simulink model "controlAerobi"  (R2017b)
settings: Solver=FixedStepDiscrete  StartTime=0.0  StopTime=inf  FixedStep=Ts  RelTol=1e-3
InitFcn:
  | load Navio2_bus;
  | Ts=0.0025;
StopFcn:
  | %save_system('controlAerobi.slx');
  | %run('D:\Eclipse_Workspaces\workspace_rasp\AutoPilot\contAerobi\UpdateFiles\CopyBuildFiles.m');
undefined symbols (not defined in the file or in its folder): DiscIntNeverNeededParam
libraries: simulink x36, sharedutil x1, sharedtransform x1, dspsigops x1
(part 4 of 4)

== matlab function controlAerobi/Sensors/position/px4fow/Liner Fixed-gain Filter1 ==
  data: thrust input; dx input; dy input; quality input; roll input; pitch input; yaw input; a_b input; vx output; vy output; ax output; ay output
function [vx,vy,ax,ay] = linear_Fixed_Gain_Filter(thrust,dx,dy,quality,roll,pitch,yaw,a_b)

dt = 0.0025;
m = 2.5;
mu = 0.87;
R_yaw = [cos(yaw) -sin(yaw);sin(yaw) cos(yaw)];
a_b = a_b/norm(a_b);
a_I = [a_b(2)-sin(pitch);
       -(a_b(1)+sin(roll)*cos(pitch));
       a_b(3)-cos(roll)*cos(pitch)];
persistent x_k P_k
if isempty(x_k)||isempty(P_k)
    x_k = [0;0];
    P_k = [1 0;0 1;];
   
else
%     if thrust < 40
%         thrust = 40;
%     elseif thrust >120
%         thrust = 120;
%     end
%     u = 62.5/thrust;
      
    x_I = [dx;dy];
    
    F = [mu/m          0;
                0   mu/m];
    
    H = [mu/m          0; 
                0   mu/m; 
                1          0;
                0          1;];
            
    Q = diag([1 1]);
    if quality >= 100
        R = diag([0.5 0.5 0.1 0.1]);
    else
        R = diag([0.5 0.5 100000 100000]);
    end
    
    z_k = [a_I(1);a_I(2);x_I(1);x_I(2)];
    y_k = x_k;
        %---------PREDICTION---------%
    %1. Project the state ahead
        x_k = F * x_k;% + B * w_k;
    %2. Project the error covariance ahead
        P_k = F * P_k * F' + Q;  
    %--------CORRECTION----------%
    %1. Compute the Kalman Gain
        K_k = P_k * H' / (H*P_k*H' + R);
        
        resid = z_k - H*y_k;
    %2. Update the estimate via measurement
        x_k = x_k + K_k * resid;
    %3. Update the error covariance
        P_k = (eye(size(K_k,1)) - K_k * H) * P_k;    
    
 
end
v = R_yaw'*x_k;
vx = v(1);
vy = v(2);
ax = a_I(1);
ay = a_I(2);

== matlab function controlAerobi/Sensors/position/EKF_total_Station_Lidar/filter/EKF2_XYZ ==
  data: x_hat output; y_hat output; z_hat output; x input; y input; z input; dx input; dy input; roll input; pitch input; yaw input; acc_ input; d_sf11 input; KQ input; KR input; a_b input; dx_hat output; dy_hat output; dz_hat output
function [x_hat,y_hat,z_hat,dx_hat,dy_hat,dz_hat] = EKF(x,y,z,dx,dy,roll,pitch,yaw,acc_,d_sf11,KQ,KR,a_b)

dt = 0.0025;
a_b = a_b/norm(a_b);
a_I = [(acc_(2)-sin(pitch))*cos(yaw)-sin(yaw)*((-acc_(1)-sin(roll)*cos(pitch)));
        sin(yaw)*(acc_(2)-sin(pitch))+cos(yaw)*((-acc_(1)-sin(roll)*cos(pitch)));
        a_b(3)-cos(roll)*cos(pitch)];

persistent  x_k P_k x0 y0 z0 
if isempty(x_k) || isempty(P_k)|| isempty(x0)|| isempty(y0)|| isempty(z0)
    x_k = [0;0;0;0;z;0];  
    P_k = eye(6,6);
    x0 = 0;
    y0 = 0;
    z0 = 0;
else
    z_corr = d_sf11*sin(roll);

    z0 = (z*cos(roll)+z_corr)*cos(pitch);
    x0 = x;
    y0 = y;
        F = [1 dt 0  0 0 0;
             0  1 0  0 0 0;
             0  0 1 dt 0 0;
             0  0 0  1 0 0;
             0  0 0  0 1 dt;
             0  0 0  0 0 1];
        B = [0.5*dt^2       0       0;
                   dt       0       0;
                   0 0.5*dt^2       0;
                   0       dt       0;
                   0       0 0.5*dt^2;
                   0       0       dt];
        w_k = [a_I(1);a_I(2);a_I(3)];        
        z_k = [x0;dx;y0;dy;z0;];
        y_k = [x_k(1);x_k(2);x_k(3);x_k(4);x_k(5);];
        H =[1   0 0  0 0  0;
            0   1 0  0 0  0;
            0   0 1  0 0  0;
            0   0 0  1 0  0;
            0   0 0  0 1  0;
            ];
        Q = diag(KQ);
        R = diag(KR);
    %---------PREDICTION---------%
    %1. Project the state ahead
        x_k = F * x_k + B * w_k;
    %2. Project the error covariance ahead
        P_k = F * P_k * F' + Q;  
    %--------CORRECTION----------%
    %1. Compute the Kalman Gain
        K_k = P_k * H' / (H*P_k*H' + R);
        
        resid = z_k - y_k;
    %2. Update the estimate via measurement
        x_k = x_k + K_k * resid;
    %3. Update the error covariance
        P_k = (eye(size(K_k,1)) - K_k * H) * P_k;    

end
x_hat = x_k(1);
y_hat = x_k(3);
z_hat = x_k(5);
dx_hat = x_k(2);
dy_hat = x_k(4);
dz_hat = x_k(6);

== matlab function controlAerobi/Sensors/control_modes/ModeBlock/enable pos ==
  data: t input; e output
function e   = enable_pos(t)

if isnan(t) || isinf(t)  || t == 0
    e = 0;
else

    e = 1;
end
